simulink model "rc_cir_5"  (R2020a)
settings: Solver=VariableStepAuto  StartTime=0.0  StopTime=10.0  RelTol=1e-3
model workspace (MAT data in the model file):
  c = Simulink.Parameter
  c.Value = 1e-05
  c.DataType = 'auto'
  c.Dimensions = [1 1]
  r = Simulink.Parameter
  r.Value = 10
  r.DataType = 'auto'
  r.Dimensions = [1 1]
libraries: simulink x2
settings Model: Creator=akhil singh  LastModifiedBy=akhil singh

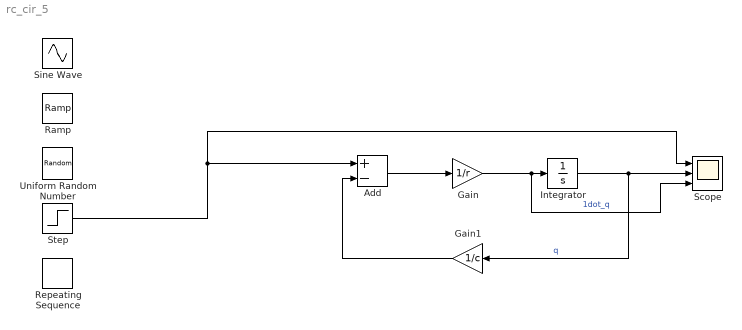
== system rc_cir_5 ==
  Add : Sum  Inputs=+-
  Gain : Gain  Gain=1/r
  Gain1 : Gain  Gain=1/c
  Integrator : Integrator
  Ramp : simulink/Sources/Ramp  slope=1  start=0  InitialOutput=0
  Repeating Sequence : simulink/Sources/Repeating Sequence  rep_seq_t=[0 2]  rep_seq_y=[0 2]
  Scope : Scope  NumInputPorts=3
  Sine Wave : Sin  SampleTime=0
  Step : Step  SampleTime=0
  Uniform Random Number : UniformRandomNumber  SampleTime=0.1
  wires:
  Add/1 -> Gain/1
  Gain/1 -> Scope/3, Integrator/1  "1dot_q"
  Integrator/1 -> Gain1/1, Scope/2  "q"
  Gain1/1 -> Add/2
  Step/1 -> Scope/1, Add/1
